simulink model "untitled"  (R2013b)
settings: Solver=ode45  StartTime=0.0  StopTime=0.04  RelTol=1e-3
libraries: powerlib_meascontrol x1
settings Model: Creator=Veronica  LastModifiedBy=Veronica

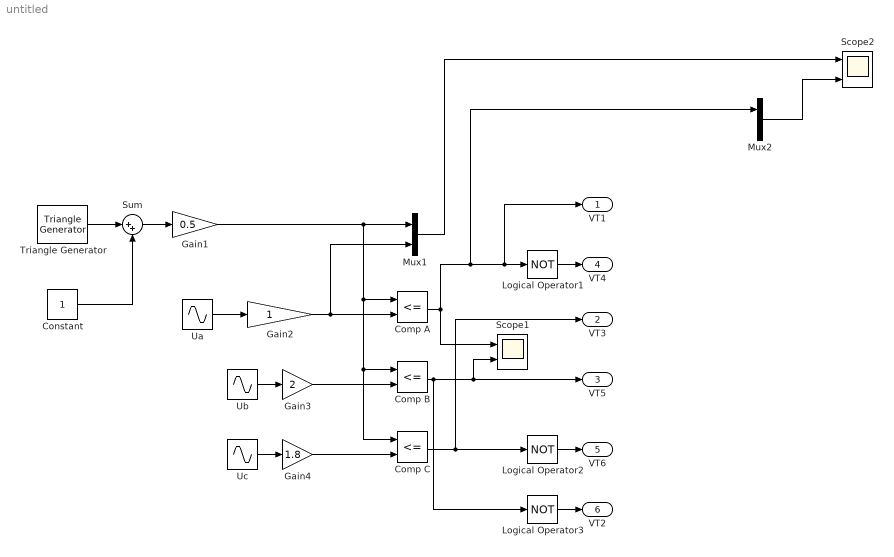
== system untitled ==
  Comp A : RelationalOperator  Operator=<=  OutDataTypeStr=boolean
  Comp B : RelationalOperator  Operator=<=  OutDataTypeStr=boolean
  Comp C : RelationalOperator  Operator=<=  OutDataTypeStr=boolean
  Constant : Constant
  Gain1 : Gain  Gain=0.5
  Gain2 : Gain
  Gain3 : Gain  Gain=2
  Gain4 : Gain  Gain=1.8
  Logical Operator1 : Logic  Operator=NOT  AllPortsSameDT=off  OutDataTypeStr=boolean
  Logical Operator2 : Logic  Operator=NOT  AllPortsSameDT=off  OutDataTypeStr=boolean
  Logical Operator3 : Logic  Operator=NOT  AllPortsSameDT=off  OutDataTypeStr=boolean
  Mux1 : Mux  Inputs=2
  Mux2 : Mux  Inputs=2
  Scope1 : Scope  NumInputPorts=2
      settings: TimeRange=0.05  YMin=-0.2~-0.2  YMax=1.2~1.2  SampleInput=on  SampleTime=1/60/5000
  Scope2 : Scope  NumInputPorts=2
      settings: TimeRange=0.01  YMin=-0.2~-0.2  YMax=1.2~1.2  SampleInput=on  SampleTime=1/60/5000
  Sum : Sum  Inputs=|++
  Triangle Generator : powerlib_meascontrol/Pulse & Signal Generators/Triangle Generator  Freq=6000  Phase=0  Ts=0
  Ua : Sin  Frequency=2*pi*50  SampleTime=0  VectorParams1D=off
  Ub : Sin  Frequency=2*pi*50  Phase=1.0472  SampleTime=0  VectorParams1D=off
  Uc : Sin  Frequency=2*pi*50  Phase=2.0944  SampleTime=0  VectorParams1D=off
  VT1 : Outport
  VT3 : Outport  Port=2
  VT5 : Outport  Port=3
  VT4 : Outport  Port=4
  VT6 : Outport  Port=5
  VT2 : Outport  Port=6
  wires:
  Uc/1 -> Gain4/1
  Ub/1 -> Gain3/1
  Ua/1 -> Gain2/1
  Logical Operator1/1 -> VT4/1
  Logical Operator2/1 -> VT6/1
  Logical Operator3/1 -> VT2/1
  Comp C/1 -> VT3/1, Logical Operator2/1
  Comp B/1 -> Logical Operator3/1, Scope1/2, VT5/1
  Gain1/1 -> Comp C/1, Comp B/1, Comp A/1, Mux1/1
  Gain2/1 -> Mux1/2, Comp A/2
  Gain3/1 -> Comp B/2
  Gain4/1 -> Comp C/2
  Mux1/1 -> Scope2/1
  Comp A/1 -> Scope1/1, Mux2/1, Logical Operator1/1, VT1/1
  Triangle Generator/1 -> Sum/1
  Constant/1 -> Sum/2
  Sum/1 -> Gain1/1
  Mux2/1 -> Scope2/2
